simulink model "toy_car"  (R2022b)
settings: Solver=ode1  StartTime=0.0  StopTime=inf  FixedStep=0.001  RelTol=1e-3
settings Model: Creator=user  LastModifiedBy=user

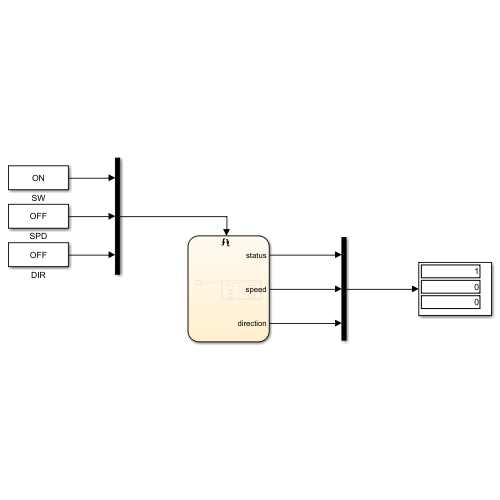
[thumbnail: Simulink's stored preview of the top-level diagram]
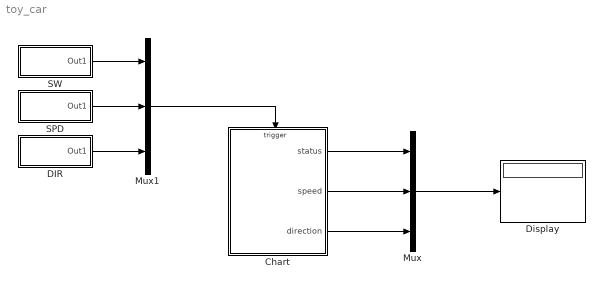
== system toy_car ==
  Chart : Stateflow chart  TreatAsAtomicUnit=on
  DIR : Subsystem  StartFcn=|  mask{str=OFF}
      | set_param(gcb, 'str', 'OFF');
      | set_param([gcb '/Constant'], 'Value', '0');
      mask prompts: str "Display name:"
      settings: OpenFcn=|
      | old_val = get_param([gcb '/Constant'], 'Value');
      | 
      | switch old_val
      | case '0'
      |     set_param(gcb, 'str', 'ON');
      |     set_param([gcb '/Constant'], 'Value', '1');
      | 
      | case '1'
      |     set_param(gcb, 'str', 'OFF');
      |     set_param([gcb '/Constant'], 'Value', '0');
      | 
      | otherwise
      |     set_param(gcb, 'str', 'ON');
      |     set_param([gcb '/Constant'], 'Value', '0');
      | 
      | end
      mask DialogControl ParameterGroupVar Prompt: 파라미터
      mask Display: disp(get_param(gcb,'str'));
  Display : Display
  Mux : Mux  Inputs=3
  Mux1 : Mux  Inputs=3
  SPD : Subsystem  StartFcn=|  mask{str=OFF}
      | set_param(gcb, 'str', 'OFF');
      | set_param([gcb '/Constant'], 'Value', '0');
      mask prompts: str "Display name:"
      settings: OpenFcn=|
      | old_val = get_param([gcb '/Constant'], 'Value');
      | 
      | switch old_val
      | case '0'
      |     set_param(gcb, 'str', 'ON');
      |     set_param([gcb '/Constant'], 'Value', '1');
      | 
      | case '1'
      |     set_param(gcb, 'str', 'OFF');
      |     set_param([gcb '/Constant'], 'Value', '0');
      | 
      | otherwise
      |     set_param(gcb, 'str', 'ON');
      |     set_param([gcb '/Constant'], 'Value', '0');
      | 
      | end
      mask DialogControl ParameterGroupVar Prompt: 파라미터
      mask Display: disp(get_param(gcb,'str'));
  SW : Subsystem  StartFcn=|  mask{str=ON}
      | set_param(gcb, 'str', 'OFF');
      | set_param([gcb '/Constant'], 'Value', '0');
      mask prompts: str "Display name:"
      settings: OpenFcn=|
      | old_val = get_param([gcb '/Constant'], 'Value');
      | 
      | switch old_val
      | case '0'
      |     set_param(gcb, 'str', 'ON');
      |     set_param([gcb '/Constant'], 'Value', '1');
      | 
      | case '1'
      |     set_param(gcb, 'str', 'OFF');
      |     set_param([gcb '/Constant'], 'Value', '0');
      | 
      | otherwise
      |     set_param(gcb, 'str', 'ON');
      |     set_param([gcb '/Constant'], 'Value', '0');
      | 
      | end
      mask DialogControl ParameterGroupVar Prompt: 파라미터
      mask Display: disp(get_param(gcb,'str'));
  wires:
  Chart/1(status) -> Mux/1
  Chart/2(speed) -> Mux/2
  Mux/1 -> Display/1
  Mux1/1 -> Chart/Trigger
  SW/1(Out1) -> Mux1/1
  SPD/1(Out1) -> Mux1/2
  DIR/1(Out1) -> Mux1/3
  Chart/3(direction) -> Mux/3

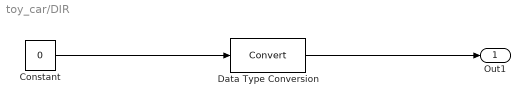
== system toy_car/DIR ==
  Constant : Constant  Value=0
  Data Type Conversion : DataTypeConversion  SaturateOnIntegerOverflow=off  RndMeth=Floor
  Out1 : Outport
  wires:
  Data Type Conversion/1 -> Out1/1
  Constant/1 -> Data Type Conversion/1

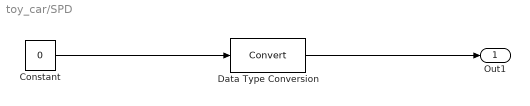
== system toy_car/SPD ==
  Constant : Constant  Value=0
  Data Type Conversion : DataTypeConversion  SaturateOnIntegerOverflow=off  RndMeth=Floor
  Out1 : Outport
  wires:
  Data Type Conversion/1 -> Out1/1
  Constant/1 -> Data Type Conversion/1

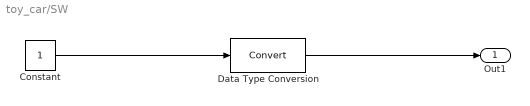
== system toy_car/SW ==
  Constant : Constant
  Data Type Conversion : DataTypeConversion  SaturateOnIntegerOverflow=off  RndMeth=Floor
  Out1 : Outport
  wires:
  Data Type Conversion/1 -> Out1/1
  Constant/1 -> Data Type Conversion/1

== stateflow chart toy_car/Chart ==
  settings: executeAtInitialization=1
  state OFF
  state ON
    state DIRECTION [parallel]
      settings: executionOrder=1
      (history)
      state FW
      state BW
      (default) -> FW : / {direction = 1}
      FW -> BW : DIR /{direction = -1;}
      BW -> FW : DIR /{direction = 1;}
    state SPEED [parallel]
      settings: executionOrder=2
      (history)
      state SLOW
      state FAST
      (default) -> SLOW : / {speed = 1}
      SLOW -> FAST : SPD /{speed = 2;}
      FAST -> SLOW : SPD /{speed = 1;}
  (default) -> OFF : / {speed = 0}
  ON -> OFF : SW /{status = 0; speed = 0, direction = 0;}
  OFF -> ON : SW /{status = 1;}
  data: status output; speed output; direction output
  events: SW input EITHER_EDGE_EVENT; SPD input EITHER_EDGE_EVENT; DIR input EITHER_EDGE_EVENT
